simulink model "omega_estimator_withKF"  (R2020a)
settings: Solver=ode23tb  StartTime=0.0  StopTime=simlength  MaxStep=Ts
values from neighbouring files (symbols this model uses):
  q1kalman = 1    [init_omega_estimator_2022_02_10.m]
  q2kalman = 100    [init_omega_estimator_2022_02_10.m]
  Rkalman = 1    [init_omega_estimator_2022_02_10.m]
  Tc = 1e-5    (= 1e-05)    [init_omega_estimator_2022_02_10.m]
  Ts = 1/1e3    (= 0.001)    [init_omega_estimator_2022_02_10.m]
  w = 2*pi*f    (= 314.159265359)    [init_omega_estimator_2022_02_10.m]
libraries: simulink x1
settings Model: SimulationMode=accelerator  Creator=dbagn  LastModifiedBy=dabagnara
settings SolverCC: SolverResetMethod=Robust
settings DataIOCC: ReturnWorkspaceOutputs=off

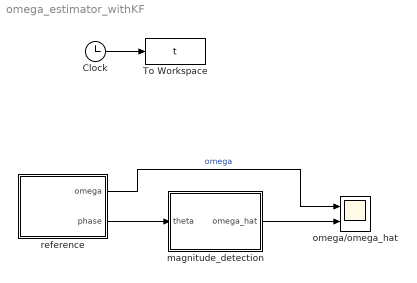
== system omega_estimator_withKF ==
  Clock : Clock
  To Workspace : ToWorkspace  VariableName=t  SampleTime=Tc
      settings: MaxDataPoints=Nc
  magnitude_detection : Subsystem
  omega/omega_hat : Scope  NumInputPorts=2
  reference : Subsystem
  wires:
  Clock/1 -> To Workspace/1
  reference/2(phase) -> magnitude_detection/1(theta)
  magnitude_detection/1(omega_hat) -> omega/omega_hat/2
  reference/1(omega) -> omega/omega_hat/1  "omega"

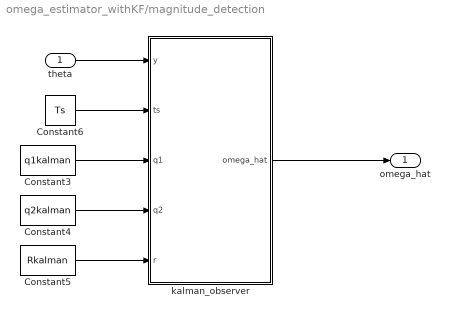
== system omega_estimator_withKF/magnitude_detection ==
  theta : Inport
  Constant3 : Constant  Value=q1kalman
  Constant4 : Constant  Value=q2kalman
  Constant5 : Constant  Value=Rkalman
  Constant6 : Constant  Value=Ts
  kalman_observer : MATLAB Function  TreatAsAtomicUnit=on  SystemSampleTime=Ts
  omega_hat : Outport
  wires:
  theta/1 -> kalman_observer/1(y)
  Constant6/1 -> kalman_observer/2(ts)
  Constant5/1 -> kalman_observer/5(r)
  Constant3/1 -> kalman_observer/3(q1)
  Constant4/1 -> kalman_observer/4(q2)
  kalman_observer/1(omega_hat) -> omega_hat/1

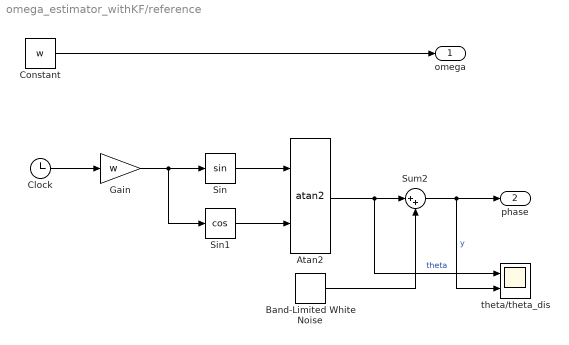
== system omega_estimator_withKF/reference ==
  Atan2 : Trigonometry  Operator=atan2
  Band-Limited White Noise : simulink/Sources/Band-Limited White Noise  Cov=Tc*0.05  Ts=Tc  seed=[23341]
  Clock : Clock
  Constant : Constant  Value=w
  Gain : Gain  Gain=w
  Sin : Trigonometry
  Sin1 : Trigonometry  Operator=cos
  Sum2 : Sum  Inputs=|++
  theta/theta_dis : Scope  NumInputPorts=2
  omega : Outport
  phase : Outport  Port=2
  wires:
  Clock/1 -> Gain/1
  Constant/1 -> omega/1
  Gain/1 -> Sin1/1, Sin/1
  Sin/1 -> Atan2/1
  Sin1/1 -> Atan2/2
  Band-Limited White Noise/1 -> Sum2/2
  Atan2/1 -> theta/theta_dis/1, Sum2/1  "theta"
  Sum2/1 -> theta/theta_dis/2, phase/1  "y"

== matlab function omega_estimator_withKF/magnitude_detection/kalman_observer ==
  data: y input; omega_hat output; ts input; q1 input; q2 input; r input
function omega_hat   = KFO(y,ts,q1,q2,r)

    persistent   x1_po x2_po p11_po p12_po p21_po p22_po

    if isempty(x1_po)
        x1_po = 0;
        x2_po = 0;
        p11_po = 0;
        p12_po = 0;
        p21_po = 0;
        p22_po = 0;        
    end
    
    a11 = 1;
    a12 = ts;
    a21 = 0;
    a22 = 1;
   
    x1_pr = a11*x1_po + a12*x2_po;
    x2_pr = a21*x1_po + a22*x2_po;
    
    x1_pr = -pi + mod(x1_pr+3*pi,2*pi);
    e = y - x1_pr;
    
    if e > pi
        e = e - 2*pi;
    end
    
    if e < -pi
        e = e + 2*pi;
    end
    
    p11_pr = q1 + a11*(a11*p11_po+a12*p21_po) + a12*(a11*p12_po+a12*p22_po);
    p12_pr = a21*(a11*p11_po+a12*p21_po) + a22*(a11*p12_po+a12*p22_po);
    p21_pr = a11*(a21*p11_po+a22*p21_po) + a12*(a21*p12_po+a22*p22_po);
    p22_pr = q2 + a21*(a21*p11_po+a22*p21_po) + a22*(a21*p12_po+a22*p22_po);
    
    l1 = p11_pr/(p11_pr + r);
    l2 = p21_pr/(p11_pr + r);
    
    x1_po = x1_pr + l1*e;
    x2_po = x2_pr + l2*e;
    
    p11_po = (1-l1)*p11_pr;
    p12_po = (1-l1)*p12_pr;
    p21_po = p21_pr-l2*p11_pr;
    p22_po = p22_pr-l2*p12_pr;
   
    omega_hat = x2_pr;
end
